simulink model "cds_hg"  (R2018a)
settings: Solver=FixedStepAuto  StartTime=0.0  StopTime=5  FixedStep=0.001  RelTol=1e-3
settings Model: Creator=DuyNam  LastModifiedBy=DuyNam
settings SolverCC: ZeroCrossAlgorithm=Adaptive
settings DebuggingCC: MaxConsecutiveZCsMsg=none

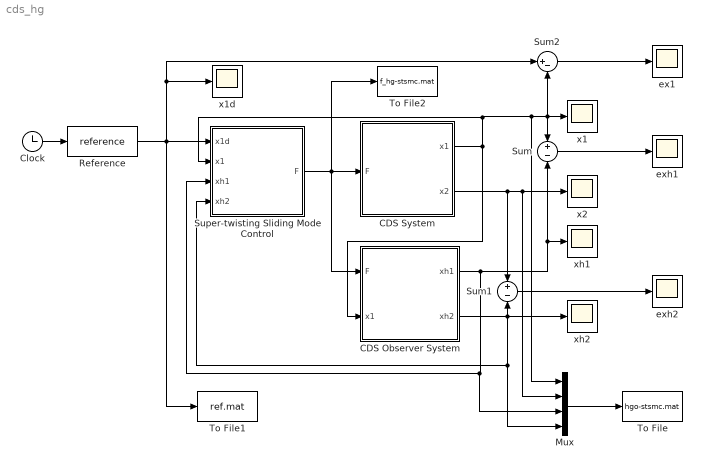
== system cds_hg ==
  CDS Observer System : Subsystem
  CDS System : Subsystem
  Clock : Clock
  Mux : Mux
  Reference : MATLABFcn  MATLABFcn=reference  OutputDimensions=4
  Sum : Sum  Inputs=+|-
  Sum1 : Sum  Inputs=+|-
  Sum2 : Sum  Inputs=|+-
  Super-twisting Sliding Mode Control : Subsystem
  To File : ToFile  Filename=hgo-stsmc.mat  SaveFormat=Timeseries
  To File1 : ToFile  Filename=ref.mat  SaveFormat=Timeseries
  To File2 : ToFile  Filename=f_hg-stsmc.mat  SaveFormat=Timeseries
  ex1 : Scope
  exh1 : Scope
  exh2 : Scope
  x1 : Scope
  x1d : Scope
  x2 : Scope
  xh1 : Scope
  xh2 : Scope
  wires:
  Super-twisting Sliding Mode Control/1(F) -> To File2/1, CDS System/1(F), CDS Observer System/1(F)
  CDS System/1(x1) -> CDS Observer System/2(x1), Super-twisting Sliding Mode Control/2(x1), Mux/1, Sum2/2, Sum/1, x1/1
  CDS System/2(x2) -> Sum1/1, Mux/2, x2/1
  CDS Observer System/2(xh2) -> Super-twisting Sliding Mode Control/4(xh2), Mux/4, Sum1/2, xh2/1
  CDS Observer System/1(xh1) -> Mux/3, Super-twisting Sliding Mode Control/3(xh1), Sum/2, xh1/1
  Sum/1 -> exh1/1
  Sum1/1 -> exh2/1
  Clock/1 -> Reference/1
  Reference/1 -> To File1/1, Sum2/1, x1d/1, Super-twisting Sliding Mode Control/1(x1d)
  Sum2/1 -> ex1/1
  Mux/1 -> To File/1

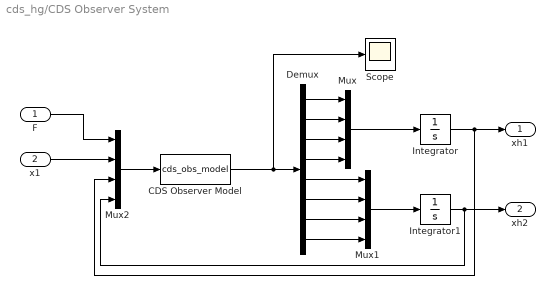
== system cds_hg/CDS Observer System ==
  F : Inport
  x1 : Inport  Port=2
  CDS Observer Model : MATLABFcn  MATLABFcn=cds_obs_model  OutputDimensions=8
  Demux : Demux  Outputs=8
  Integrator : Integrator  InitialCondition=[0;0;0;0]
  Integrator1 : Integrator  InitialCondition=[0;0;0;0]
  Mux : Mux
  Mux1 : Mux
  Mux2 : Mux
  Scope : Scope
  xh1 : Outport
  xh2 : Outport  Port=2
  wires:
  Demux/6 -> Mux1/2
  Demux/3 -> Mux/3
  Integrator1/1 -> xh2/1, Mux2/4
  Demux/4 -> Mux/4
  CDS Observer Model/1 -> Scope/1, Demux/1
  Integrator/1 -> xh1/1, Mux2/3
  Demux/8 -> Mux1/4
  Mux1/1 -> Integrator1/1
  Demux/1 -> Mux/1
  Demux/7 -> Mux1/3
  Mux/1 -> Integrator/1
  Demux/5 -> Mux1/1
  x1/1 -> Mux2/2
  Mux2/1 -> CDS Observer Model/1
  Demux/2 -> Mux/2
  F/1 -> Mux2/1

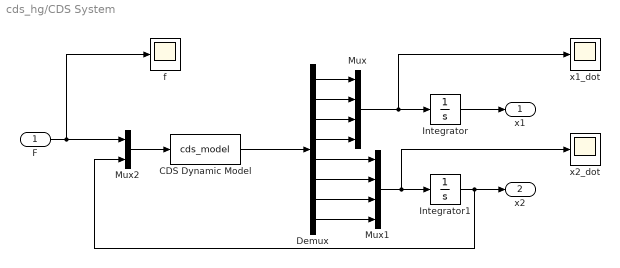
== system cds_hg/CDS System ==
  F : Inport
  CDS Dynamic Model : MATLABFcn  MATLABFcn=cds_model  OutputDimensions=8
  Demux : Demux  Outputs=8
  Integrator : Integrator  InitialCondition=[0.5;0.5;0.5;0]
  Integrator1 : Integrator  InitialCondition=[0;0;0;0]
  Mux : Mux
  Mux1 : Mux
  Mux2 : Mux  Inputs=2
  f : Scope
  x1_dot : Scope
  x2_dot : Scope
  x1 : Outport
  x2 : Outport  Port=2
  wires:
  Demux/7 -> Mux1/3
  Demux/5 -> Mux1/1
  Demux/2 -> Mux/2
  Mux2/1 -> CDS Dynamic Model/1
  Mux/1 -> x1_dot/1, Integrator/1
  Integrator1/1 -> x2/1, Mux2/2
  Demux/1 -> Mux/1
  Demux/4 -> Mux/4
  Demux/3 -> Mux/3
  Demux/8 -> Mux1/4
  Demux/6 -> Mux1/2
  Mux1/1 -> x2_dot/1, Integrator1/1
  CDS Dynamic Model/1 -> Demux/1
  F/1 -> f/1, Mux2/1
  Integrator/1 -> x1/1

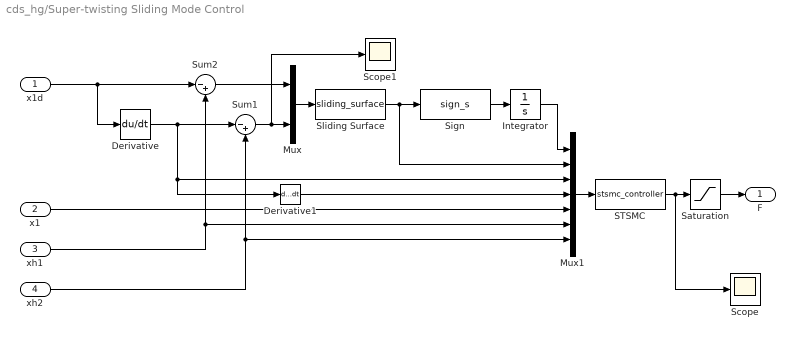
== system cds_hg/Super-twisting Sliding Mode Control ==
  x1d : Inport
  x1 : Inport  Port=2
  xh1 : Inport  Port=3
  xh2 : Inport  Port=4
  Derivative : Derivative
  Derivative1 : Derivative
  Integrator : Integrator  InitialCondition=[0;0;0;0]
  Mux : Mux  Inputs=2
  Mux1 : Mux  Inputs=7
  STSMC : MATLABFcn  MATLABFcn=stsmc_controller  OutputDimensions=4
  Saturation : Saturate  UpperLimit=[200;200;200;inf]  LowerLimit=-[200;200;200;inf]
  Scope : Scope
  Scope1 : Scope
  Sign : MATLABFcn  MATLABFcn=sign_s  OutputDimensions=4
  Sliding Surface : MATLABFcn  MATLABFcn=sliding_surface  OutputDimensions=4
  Sum1 : Sum  Inputs=|-+
  Sum2 : Sum  Inputs=|-+
  F : Outport
  wires:
  x1d/1 -> Derivative/1, Sum2/1
  Derivative/1 -> Derivative1/1, Mux1/3, Sum1/1
  xh1/1 -> Mux1/6, Sum2/2
  xh2/1 -> Mux1/7, Sum1/2
  Sum2/1 -> Mux/1
  Sum1/1 -> Scope1/1, Mux/2
  Mux/1 -> Sliding Surface/1
  Sliding Surface/1 -> Sign/1, Mux1/2
  Mux1/1 -> STSMC/1
  Integrator/1 -> Mux1/1
  Derivative1/1 -> Mux1/4
  x1/1 -> Mux1/5
  Sign/1 -> Integrator/1
  STSMC/1 -> Scope/1, Saturation/1
  Saturation/1 -> F/1
